simulink model "model"  (R2015a)
settings: Solver=ode45  StartTime=0.0  StopTime=20.0  RelTol=1e-3
settings Model: Creator=yusuke  LastModifiedBy=yusuke

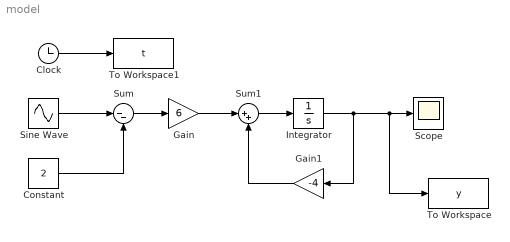
== system model ==
  Clock : Clock
  Constant : Constant  Value=2
  Gain : Gain  Gain=6
  Gain1 : Gain  Gain=-4
  Integrator : Integrator  InitialCondition=-5
  Scope : Scope
      settings: TimeRange=40  YMin=-2.967952127659574  YMax=-1.567952127659574
  Sine Wave : Sin  SampleTime=0.01
  Sum : Sum  Inputs=|--
  Sum1 : Sum  Inputs=|++
  To Workspace : ToWorkspace  VariableName=y  SaveFormat=Structure With Time  SampleTime=-1
  To Workspace1 : ToWorkspace  VariableName=t  SaveFormat=Structure With Time  SampleTime=-1
  wires:
  Sine Wave/1 -> Sum/1
  Constant/1 -> Sum/2
  Sum/1 -> Gain/1
  Gain/1 -> Sum1/1
  Sum1/1 -> Integrator/1
  Gain1/1 -> Sum1/2
  Integrator/1 -> To Workspace/1, Scope/1, Gain1/1
  Clock/1 -> To Workspace1/1
